simulink model "AVoWk3Prob1and2"  (R2021b)
settings: Solver=FixedStepAuto  StartTime=0.0  StopTime=10.0  FixedStep=0.01  RelTol=1e-3
values from neighbouring files (symbols this model uses):
  a = 2    [AndyVoLab2.m]    (also in ME4391L_LAB2_Goulenko_P2.m)
  b = 3    [AndyVoLab2.m]    (also in ME4391L_LAB2_Goulenko_P2.m)
  c = 0.25    [AndyVoLab2.m]    (also in ME4391L_LAB2_Goulenko_P2.m)
  d = 1 * 2*pi    (= 6.28318530718)    [AndyVoLab2.m]    (also in ME4391L_LAB2_Goulenko_P2.m)
settings Model: Creator=andyvo  LastModifiedBy=andyvo

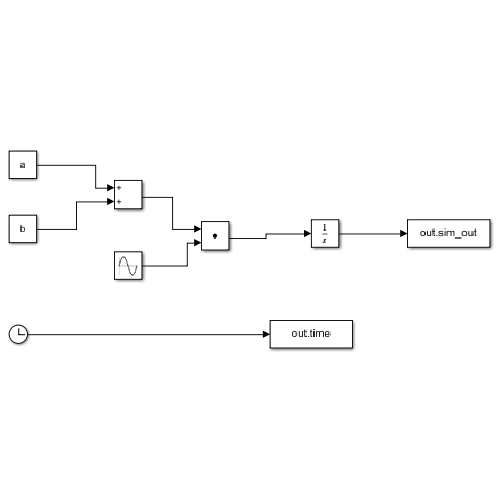
[thumbnail: Simulink's stored preview of the top-level diagram]
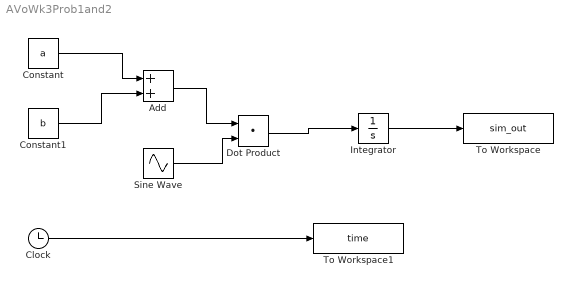
== system AVoWk3Prob1and2 ==
  Add : Sum
  Clock : Clock
  Constant : Constant  Value=a
  Constant1 : Constant  Value=b
  Dot Product : DotProduct  InputSameDT=on  OutDataTypeStr=Inherit: Inherit via internal rule
  Integrator : Integrator
  Sine Wave : Sin  Amplitude=c  Frequency=d  SampleTime=0
  To Workspace : ToWorkspace  VariableName=sim_out  SampleTime=-1
  To Workspace1 : ToWorkspace  VariableName=time  SampleTime=-1
  wires:
  Constant1/1 -> Add/2
  Constant/1 -> Add/1
  Add/1 -> Dot Product/1
  Sine Wave/1 -> Dot Product/2
  Dot Product/1 -> Integrator/1
  Integrator/1 -> To Workspace/1
  Clock/1 -> To Workspace1/1
